simulink library "csc_mum_mems_unit_model_lib"  (R2014b)
settings: Solver=ode45  SolverMode=SingleTasking  StartTime=0.0  StopTime=10.0  RelTol=1e-3
values from neighbouring files (symbols this model uses):
  mnm_accel_range = 16*9.81    (= 156.96)    [csu_mnm_mems_noise_model_init.m]
  mnm_gyro_range = 250*pi/180    (= 4.36332312999)    [csu_mnm_mems_noise_model_init.m]
undefined symbols (not defined in the file): mum1_accel_bias_seed, mum1_accel_noise_seed, mum1_dcm, mum1_gyro_bias_seed, mum1_gyro_noise_seed, mum1_position
libraries: util_info_lib x1, csu_imk_imu_kinematis_lib x1, csu_mnm_mems_noise_model_lib x1
settings Model: Creator=hcannon  LastModifiedBy=Mark Agbayani

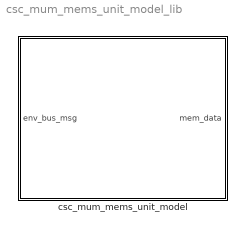
== system csc_mum_mems_unit_model_lib ==
  csc_mum_mems_unit_model : Subsystem  mask{my_imu_position=mum1_position, my_imu_dcm=mum1_dcm, my_accel_seed_v=mum1_accel_noise_seed, my_accel_bias_seed_v=mum1_accel_bias_seed, my_gyro_seed_v=mum1_gyro_noise_seed, my_gyro_bias_seed_v=mum1_gyro_bias_seed}
      mask prompts: my_imu_position "IMU Position in Body Frame"; my_imu_dcm "IMU Orientation in Body Frame"; my_accel_seed_v "Accel Output Noise Seed vector [1 x 3]"; my_accel_bias_seed_v "Accel Bias Noise Seed vector [1 x ]"; my_gyro_seed_v "Gyro Output Noise Seed vector [1 x 3]"; my_gyro_bias_seed_v "Gyro Bias Noise Seed vector [1 x 3]"

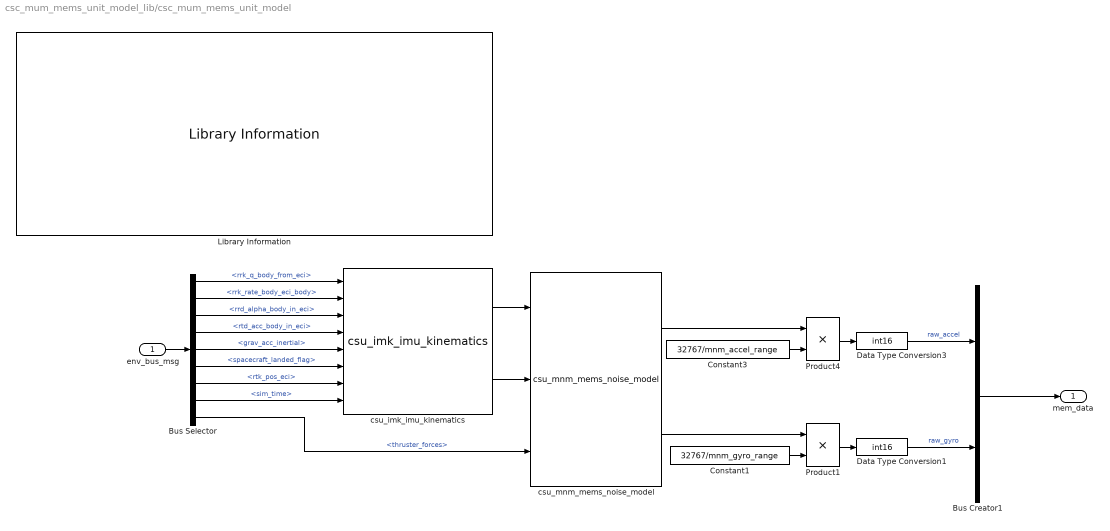
== system csc_mum_mems_unit_model_lib/csc_mum_mems_unit_model ==
  env_bus_msg : Inport
  Bus Creator1 : BusCreator  Inputs=2  NonVirtualBus=on
  Bus Selector : BusSelector  OutputSignals=lander_state_bus.rrk_q_body_from_eci,lander_state_bus.rrk_rate_body_eci_body,lander_state_bus.rrd_alpha_body_in_eci,lander_state_bus.rtd_acc_body_in_eci,enf_force_torque_msg.grav_acc_inertial,lander_state_bus.spacecraft_landed_flag,lander_state_bus.rtk_pos_eci,sim_time,actuator_msg.thruster_forces
  Constant1 : Constant  Value=32767/mnm_gyro_range  OutDataTypeStr=double
  Constant3 : Constant  Value=32767/mnm_accel_range  OutDataTypeStr=double
  Data Type Conversion1 : DataTypeConversion  OutDataTypeStr=int16  RndMeth=Round
  Data Type Conversion3 : DataTypeConversion  OutDataTypeStr=int16  RndMeth=Round
  Library Information : util_info_lib/Library Information  owner='NONE'
  Product1 : Product  RndMeth=Zero
  Product4 : Product  OutDataTypeStr=double  RndMeth=Zero
  csu_imk_imu_kinematics : csu_imk_imu_kinematis_lib/csu_imk_imu_kinematics  imu_position=my_imu_position  imu_dcm=my_imu_dcm
  csu_mnm_mems_noise_model : csu_mnm_mems_noise_model_lib/csu_mnm_mems_noise_model  accel_seed_v=my_accel_seed_v  accel_bias_seed_v=my_accel_bias_seed_v  gyro_seed_v=my_gyro_seed_v  gyro_bias_seed_v=my_gyro_bias_seed_v
  mem_data : Outport
  wires:
  Bus Selector/9 -> csu_mnm_mems_noise_model/3  "<thruster_forces>"
  Bus Selector/8 -> csu_imk_imu_kinematics/8  "<sim_time>"
  Bus Selector/7 -> csu_imk_imu_kinematics/7  "<rtk_pos_eci>"
  Bus Selector/6 -> csu_imk_imu_kinematics/6  "<spacecraft_landed_flag>"
  env_bus_msg/1 -> Bus Selector/1
  Bus Selector/1 -> csu_imk_imu_kinematics/1  "<rrk_q_body_from_eci>"
  Data Type Conversion3/1 -> Bus Creator1/1  "raw_accel"
  Bus Selector/5 -> csu_imk_imu_kinematics/5  "<grav_acc_inertial>"
  Bus Selector/4 -> csu_imk_imu_kinematics/4  "<rtd_acc_body_in_eci>"
  Bus Selector/3 -> csu_imk_imu_kinematics/3  "<rrd_alpha_body_in_eci>"
  Bus Selector/2 -> csu_imk_imu_kinematics/2  "<rrk_rate_body_eci_body>"
  Bus Creator1/1 -> mem_data/1
  csu_imk_imu_kinematics/2 -> csu_mnm_mems_noise_model/2
  csu_imk_imu_kinematics/1 -> csu_mnm_mems_noise_model/1
  csu_mnm_mems_noise_model/1 -> Product4/1
  Constant3/1 -> Product4/2
  Product4/1 -> Data Type Conversion3/1
  csu_mnm_mems_noise_model/2 -> Product1/1
  Constant1/1 -> Product1/2
  Product1/1 -> Data Type Conversion1/1
  Data Type Conversion1/1 -> Bus Creator1/2  "raw_gyro"
